simulink model "Learning_project_2"  (R2021a)
settings: Solver=VariableStepAuto  StartTime=0.0  StopTime=10.0  RelTol=1e-3
undefined symbols (not defined in the file): X
settings Model: Creator=tanmoyera  LastModifiedBy=tanmoyera

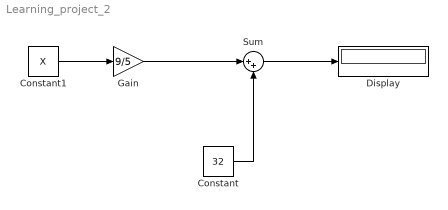
== system Learning_project_2 ==
  Constant : Constant  Value=32
  Constant1 : Constant  Value=X
  Display : Display
  Gain : Gain  Gain=9/5
  Sum : Sum  Inputs=|++
  wires:
  Constant/1 -> Sum/2
  Gain/1 -> Sum/1
  Constant1/1 -> Gain/1
  Sum/1 -> Display/1
